simulink library "mdderslib_discrete"  (Simulink 7.8)
settings: Solver=ode45  StartTime=0.0  StopTime=10.0  RelTol=1e-3
undefined symbols (not defined in the file or in its folder): DiscIntNeverNeededParam, Ts
libraries: mdderslib_discrete x3
settings Model: Creator=bures  LastModifiedBy=bures

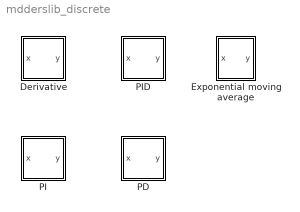
== system mdderslib_discrete ==
  Derivative : Subsystem  mask{Ts=Ts, Fa=0.5}
      mask prompts: Ts "Period"; Fa "Filter coeffiecient"
      mask Display:
      | disp('D');
      | port_label('input', 1, '');
      | port_label('output', 1, '');
  Exponential moving average : Subsystem  mask{alpha=0.5}
      mask Display:
      | disp('EMA');
      | port_label('input', 1, '');
      | port_label('output', 1, '');
  PD : Subsystem  mask{Kp=1, Kd=0, Smax=100, Smin=-100, Ts=Ts, Dmax=100, Dmin=-100}
      mask prompts: Kp "Proportional gain"; Kd "Derivative gain"; Smax "Saturation - max"; Smin "Saturation - min"; Ts "Period"; Dmax "Derivative Saturation - max"; Dmin "Derivative Saturation - min"
      mask Display:
      | disp('PD');
      | port_label('input', 1, '');
      | port_label('output', 1, '');
  PI : Subsystem  mask{Kp=1, Ki=1, Smax=100, Smin=-100, Ts=Ts, Imax=50, Imin=-50}
      mask prompts: Kp "Proportional gain"; Ki "Integral gain"; Smax "Saturation - max"; Smin "Saturation - min"; Ts "Period"; Imax "Integer Saturation - max"; Imin "Integer Saturation - min"
      mask Display:
      | disp('PI');
      | port_label('input', 1, '');
      | port_label('output', 1, '');
  PID : Subsystem  mask{Kp=1, Ki=0, Kd=0, Smax=inf, Smin=-inf, Ts=Ts, Imax=inf, Imin=-inf, Dmax=inf, Dmin=-inf}
      mask prompts: Kp "Proportional gain"; Ki "Integral gain"; Kd "Derivative gain"; Smax "Saturation - max"; Smin "Saturation - min"; Ts "Period"; Imax "Integer Saturation - max"; Imin "Integer Saturation - min"; Dmax "Derivative Saturation - max"; Dmin "Derivative Saturation - min"
      mask Display:
      | disp('PID');
      | port_label('input', 1, '');
      | port_label('output', 1, '');

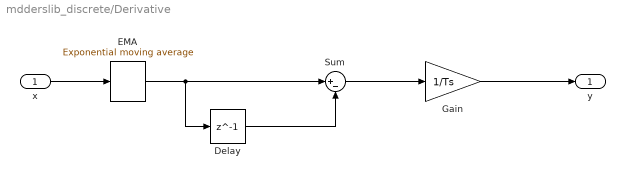
== system mdderslib_discrete/Derivative ==
  x : Inport
  Delay : Delay  DelayLength=1
  EMA : mdderslib_discrete/Exponential moving average  alpha=Fa
  Gain : Gain  Gain=1/Ts  OutDataTypeStr=Inherit: Same as input
  Sum : Sum  Inputs=|+-
  y : Outport
  wires:
  Delay/1 -> Sum/2
  x/1 -> EMA/1
  Sum/1 -> Gain/1
  Gain/1 -> y/1
  EMA/1 -> Sum/1, Delay/1

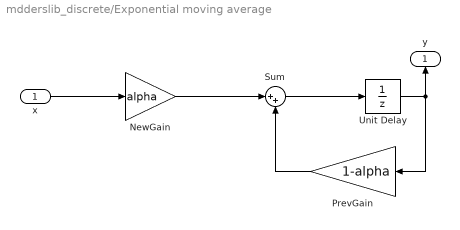
== system mdderslib_discrete/Exponential moving average ==
  x : Inport
  NewGain : Gain  Gain=alpha  OutDataTypeStr=Inherit: Same as input
  PrevGain : Gain  Gain=1-alpha  OutDataTypeStr=Inherit: Same as input
  Sum : Sum  Inputs=|++
  Unit Delay : UnitDelay  SampleTime=-1
  y : Outport
  wires:
  NewGain/1 -> Sum/1
  PrevGain/1 -> Sum/2
  Sum/1 -> Unit Delay/1
  Unit Delay/1 -> PrevGain/1, y/1
  x/1 -> NewGain/1

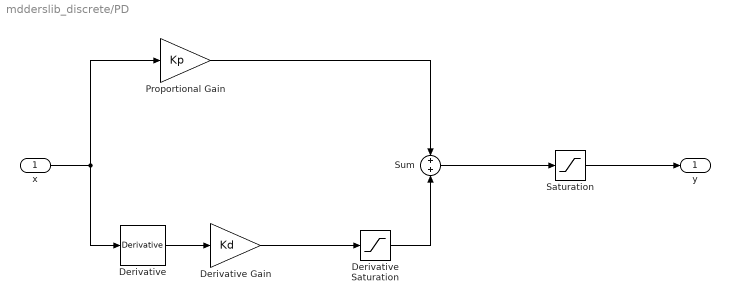
== system mdderslib_discrete/PD ==
  x : Inport
  Derivative : mdderslib_discrete/Derivative  Ts=Ts  Fa=0.5
  Derivative Saturation : Saturate  UpperLimit=Dmax  LowerLimit=Dmin
  Derivative Gain : Gain  DisableCoverage=on  Gain=Kd  OutDataTypeStr=Inherit: Same as input
  Proportional Gain : Gain  DisableCoverage=on  Gain=Kp  OutDataTypeStr=Inherit: Same as input
  Saturation : Saturate  UpperLimit=Smax  LowerLimit=Smin  LinearizeAsGain=off
  Sum : Sum  DisableCoverage=on  Inputs=+|+
  y : Outport
  wires:
  Derivative Saturation/1 -> Sum/2
  Derivative Gain/1 -> Derivative Saturation/1
  Derivative/1 -> Derivative Gain/1
  Sum/1 -> Saturation/1
  Saturation/1 -> y/1
  Proportional Gain/1 -> Sum/1
  x/1 -> Derivative/1, Proportional Gain/1

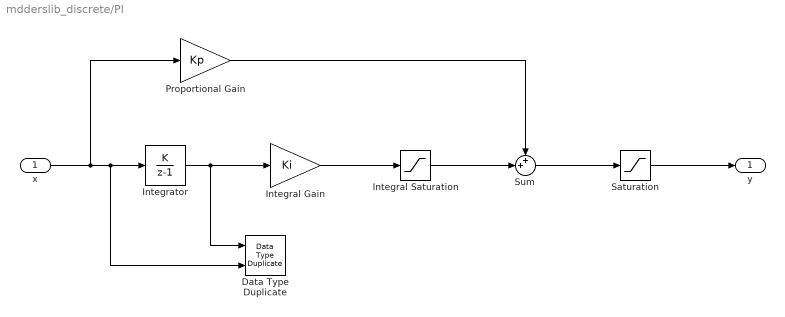
== system mdderslib_discrete/PI ==
  x : Inport
  Data Type Duplicate : DataTypeDuplicate
  Integral Saturation : Saturate  UpperLimit=Imax  LowerLimit=Imin
  Integral Gain : Gain  DisableCoverage=on  Gain=Ki  OutDataTypeStr=Inherit: Same as input
  Integrator : DiscreteIntegrator  DisableCoverage=on  IntegratorMethod=Accumulation: Forward Euler  gainval=Ts  InitialConditionMode=State only (most efficient)  SampleTime=-1  OutDataTypeStr=Inherit: Inherit via back propagation  ICPrevOutput=DiscIntNeverNeededParam  ICPrevScaledInput=DiscIntNeverNeededParam
  Proportional Gain : Gain  DisableCoverage=on  Gain=Kp  OutDataTypeStr=Inherit: Same as input
  Saturation : Saturate  UpperLimit=Smax  LowerLimit=Smin  LinearizeAsGain=off
  Sum : Sum  DisableCoverage=on  Inputs=++|
  y : Outport
  wires:
  Integral Saturation/1 -> Sum/2
  Integral Gain/1 -> Integral Saturation/1
  Integrator/1 -> Data Type Duplicate/1, Integral Gain/1
  Sum/1 -> Saturation/1
  Saturation/1 -> y/1
  Proportional Gain/1 -> Sum/1
  x/1 -> Data Type Duplicate/2, Integrator/1, Proportional Gain/1

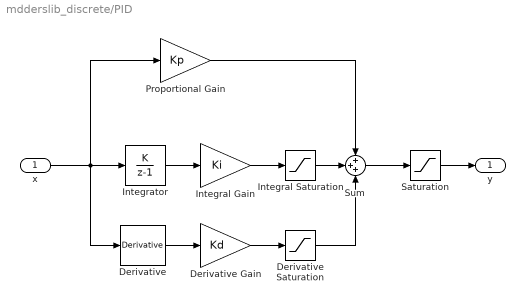
== system mdderslib_discrete/PID ==
  x : Inport
  Derivative : mdderslib_discrete/Derivative  Ts=Ts  Hs=1  Fa=0.5
  Derivative Saturation : Saturate  UpperLimit=Dmax  LowerLimit=Dmin
  Derivative Gain : Gain  DisableCoverage=on  Gain=Kd
  Integral Saturation : Saturate  UpperLimit=Imax  LowerLimit=Imin
  Integral Gain : Gain  DisableCoverage=on  Gain=Ki
  Integrator : DiscreteIntegrator  DisableCoverage=on  IntegratorMethod=Accumulation: Forward Euler  gainval=Ts  InitialConditionMode=State only (most efficient)  SampleTime=-1  ICPrevOutput=DiscIntNeverNeededParam  ICPrevScaledInput=DiscIntNeverNeededParam
  Proportional Gain : Gain  DisableCoverage=on  Gain=Kp
  Saturation : Saturate  UpperLimit=Smax  LowerLimit=Smin  LinearizeAsGain=off
  Sum : Sum  DisableCoverage=on  Inputs=+++
  y : Outport
  wires:
  x/1 -> Proportional Gain/1, Derivative/1, Integrator/1
  Proportional Gain/1 -> Sum/1
  Saturation/1 -> y/1
  Sum/1 -> Saturation/1
  Integrator/1 -> Integral Gain/1
  Integral Gain/1 -> Integral Saturation/1
  Integral Saturation/1 -> Sum/2
  Derivative/1 -> Derivative Gain/1
  Derivative Gain/1 -> Derivative Saturation/1
  Derivative Saturation/1 -> Sum/3
